simulink model "gm_nrhdlSignalDetection"  (R2023b)
settings: Solver=FixedStepDiscrete  StartTime=0.0  StopTime=sl_in.stopTime  RelTol=1e-3
undefined symbols (not defined in the file or in its folder): sl_in
libraries: hdlmdlgenlib x9, hdlsllib x5, simulink x4, dsphdlfiltering2 x4, dspsrcs4 x3, whdlmod x1
(part 1 of 2)
settings Model: SimulationMode=accelerator  Creator=The MathWorks, Inc.  LastModifiedBy=kgonipati
settings OptimizationCC: BlockReduction=off  ConditionallyExecuteInputs=off  DefaultParameterBehavior=Inlined  InheritOutputTypeSmallerThanSingle=on  ReuseModelBlockBuffer=off
settings DebuggingCC: AlgebraicLoopMsg=error  InheritedTsInSrcMsg=none  SingleTaskRateTransMsg=error  SubsystemReferenceDiagnosticForUnitTest=warning
settings HardwareCC: ProdBitPerPointer=32  ProdBitPerSizeT=32  ProdBitPerPtrDiffT=32  ProdLargestAtomicFloat=None  ProdIntDivRoundTo=Undefined  ProdEndianess=Unspecified  ProdWordSize=32  ProdHWDeviceType=ASIC/FPGA->ASIC/FPGA  TargetBitPerPointer=64  TargetBitPerSizeT=64  TargetBitPerPtrDiffT=64  TargetLongLongMode=on  TargetIntDivRoundTo=Zero  TargetEndianess=LittleEndian  TargetWordSize=64  TargetHWDeviceType=Custom Processor->MATLAB Host Computer  ProdEqTarget=off

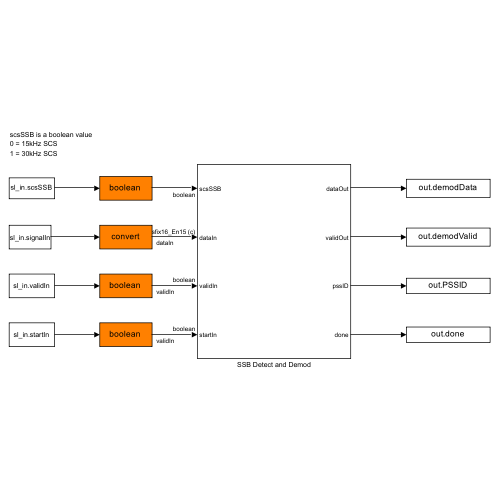
[thumbnail: Simulink's stored preview of the top-level diagram]
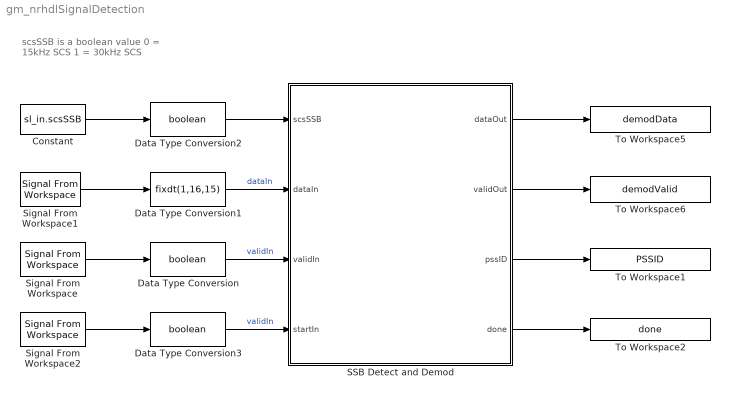
== system gm_nrhdlSignalDetection ==
  note: scsSSB is a boolean value
      | 0 = 15kHz SCS
      | 1 = 30kHz SCS
  Constant : Constant  Value=sl_in.scsSSB  SampleTime=sl_in.sampleTime
  Data Type Conversion : DataTypeConversion  OutDataTypeStr=boolean  SaturateOnIntegerOverflow=off  RndMeth=Floor
  Data Type Conversion1 : DataTypeConversion  OutDataTypeStr=fixdt(1,16,15)  RndMeth=Round  SaturateOnIntegerOverflow=off
  Data Type Conversion2 : DataTypeConversion  OutDataTypeStr=boolean  SaturateOnIntegerOverflow=off  RndMeth=Floor
  Data Type Conversion3 : DataTypeConversion  OutDataTypeStr=boolean  SaturateOnIntegerOverflow=off  RndMeth=Floor
  SSB Detect and Demod : Subsystem
  Signal From Workspace : dspsrcs4/Signal From Workspace  X=sl_in.validIn  Ts=sl_in.sampleTime  nsamps=1  OutputAfterFinalValue=Setting to zero  ignoreOrWarnInputAndFrameLengths=off  OutputFrames=off
  Signal From Workspace1 : dspsrcs4/Signal From Workspace  X=sl_in.signalIn  Ts=sl_in.sampleTime  nsamps=1  OutputAfterFinalValue=Setting to zero  ignoreOrWarnInputAndFrameLengths=off  OutputFrames=off
  Signal From Workspace2 : dspsrcs4/Signal From Workspace  X=sl_in.startIn  Ts=sl_in.sampleTime  nsamps=1  OutputAfterFinalValue=Setting to zero  ignoreOrWarnInputAndFrameLengths=off  OutputFrames=off
  To Workspace1 : ToWorkspace  VariableName=PSSID  SampleTime=-1
      settings: Save2DSignal=2-D array (concatenate along first dimension)
  To Workspace2 : ToWorkspace  VariableName=done  SampleTime=-1
      settings: Save2DSignal=2-D array (concatenate along first dimension)
  To Workspace5 : ToWorkspace  VariableName=demodData  SampleTime=-1
      settings: Save2DSignal=2-D array (concatenate along first dimension)
  To Workspace6 : ToWorkspace  VariableName=demodValid  SampleTime=-1
      settings: Save2DSignal=2-D array (concatenate along first dimension)
  wires:
  SSB Detect and Demod/4(done) -> To Workspace2/1
  Data Type Conversion3/1 -> SSB Detect and Demod/4(startIn)  "validIn"
  Signal From Workspace2/1 -> Data Type Conversion3/1
  Data Type Conversion2/1 -> SSB Detect and Demod/1(scsSSB)
  SSB Detect and Demod/3(pssID) -> To Workspace1/1
  Constant/1 -> Data Type Conversion2/1
  Data Type Conversion1/1 -> SSB Detect and Demod/2(dataIn)  "dataIn"
  SSB Detect and Demod/2(validOut) -> To Workspace6/1
  SSB Detect and Demod/1(dataOut) -> To Workspace5/1
  Data Type Conversion/1 -> SSB Detect and Demod/3(validIn)  "validIn"
  Signal From Workspace/1 -> Data Type Conversion/1
  Signal From Workspace1/1 -> Data Type Conversion1/1

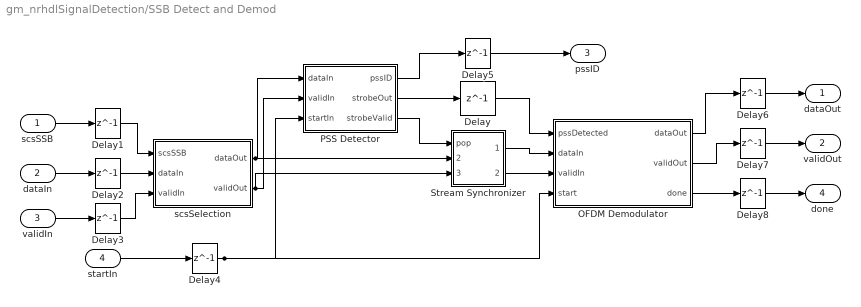
== system gm_nrhdlSignalDetection/SSB Detect and Demod ==
  scsSSB : Inport  OutDataTypeStr=boolean  PortDimensions=1  SampleTime=1.62760416666667e-08
  dataIn : Inport  Port=2  OutDataTypeStr=fixdt(1, 16, 15)  PortDimensions=1  SampleTime=1.62760416666667e-08
      settings: SignalType=complex
  validIn : Inport  Port=3  OutDataTypeStr=boolean  PortDimensions=1  SampleTime=1.62760416666667e-08
  startIn : Inport  Port=4  OutDataTypeStr=boolean  PortDimensions=1  SampleTime=1.62760416666667e-08
  Delay{,1..8} (9 alike) : Delay  DelayLength=1
  OFDM Demodulator : Subsystem
  PSS Detector : Subsystem
  Stream Synchronizer : Subsystem  mask{depth=double(512)}
  scsSelection : Subsystem
  dataOut : Outport  SampleTime=1.62760416666667e-08
  validOut : Outport  Port=2  SampleTime=1.62760416666667e-08
  pssID : Outport  Port=3  SampleTime=1.62760416666667e-08
  done : Outport  Port=4  SampleTime=1.62760416666667e-08
  wires:
  Delay1/1 -> scsSelection/1(scsSSB)
  scsSSB/1 -> Delay1/1
  Delay2/1 -> scsSelection/2(dataIn)
  dataIn/1 -> Delay2/1
  Delay3/1 -> scsSelection/3(validIn)
  validIn/1 -> Delay3/1
  scsSelection/1(dataOut) -> Stream Synchronizer/2(dataIn), PSS Detector/1(dataIn)
  startIn/1 -> Delay4/1
  scsSelection/2(validOut) -> Stream Synchronizer/3(push), PSS Detector/2(validIn)
  Delay4/1 -> OFDM Demodulator/4(start), PSS Detector/3(startIn)
  PSS Detector/1(pssID) -> Delay5/1
  PSS Detector/2(strobeOut) -> Delay/1
  PSS Detector/3(strobeValid) -> Stream Synchronizer/1(pop)
  Delay5/1 -> pssID/1
  Delay/1 -> OFDM Demodulator/1(pssDetected)
  Stream Synchronizer/2(validOut) -> OFDM Demodulator/3(validIn)
  Stream Synchronizer/1(dataOut) -> OFDM Demodulator/2(dataIn)
  OFDM Demodulator/1(dataOut) -> Delay6/1
  OFDM Demodulator/2(validOut) -> Delay7/1
  OFDM Demodulator/3(done) -> Delay8/1
  Delay6/1 -> dataOut/1
  Delay7/1 -> validOut/1
  Delay8/1 -> done/1

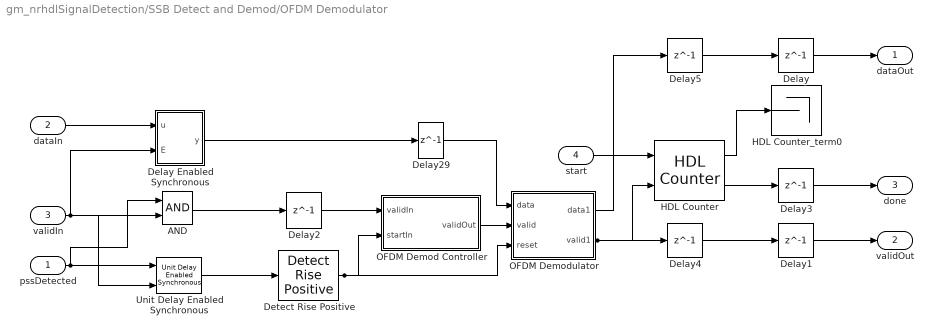
== system gm_nrhdlSignalDetection/SSB Detect and Demod/OFDM Demodulator ==
  pssDetected : Inport  OutDataTypeStr=boolean  PortDimensions=1  SampleTime=1.62760416666667e-08
  dataIn : Inport  Port=2  OutDataTypeStr=fixdt(1, 16, 15)  PortDimensions=1  SampleTime=1.62760416666667e-08
      settings: SignalType=complex
  validIn : Inport  Port=3  OutDataTypeStr=boolean  PortDimensions=1  SampleTime=1.62760416666667e-08
  start : Inport  Port=4  OutDataTypeStr=boolean  PortDimensions=1  SampleTime=1.62760416666667e-08
  AND : Logic  AllPortsSameDT=off  OutDataTypeStr=boolean
  Delay{,1..5,29} (7 alike) : Delay  DelayLength=1
  Delay Enabled Synchronous : Subsystem  mask(Delay Enabled){DelayLength=256+18, InitialCondition=0.0}
      mask prompts: DelayLength "Simulink:blkprm_prompts:DelayBlkDelayLength"; InitialCondition "Simulink:blkprm_prompts:DelayBlkInitCond"
      mask help: Implements a delay with synchronous enable.
      mask Display:
      | port_label('input', 1, 'u');
      | port_label('input', 2, 'E');
      | text(0.45,0.45, 'Z');
      | DelayLengthStr = get_param(gcbh,'DelayLength');
      | try
      |     DelayLength = eval(DelayLengthStr);
      |     text(0.55,0.55, sprintf('-%d',DelayLength));
      | catch ME
      |     text(0.55,0.55, '-N');
      | end
  Detect Rise Positive : simulink/Logic and Bit Operations/Detect Rise Positive  vinit=0  OutDataTypeStr=boolean
  HDL Counter : hdlsllib/Sources/HDL Counter  CountType=Count limited  CountInit=0  CountStep=1  CountMax=960  CountFromType=Initial value  CountFrom=0  CountResetPort=on  CountLoadPort=off  CountEnbPort=on  CountDirPort=off  CountHitOutputPort=on  CountDataType=Unsigned  CountWordLen=12  CountFracLen=0  CountSampTime=1
  HDL Counter_term0 : Terminator
  OFDM Demod Controller : Subsystem
  OFDM Demodulator : Subsystem
  Unit Delay Enabled Synchronous : hdlsllib/Discrete/Unit Delay Enabled Synchronous  InitialCondition=0.0  SampleTime=-1
  dataOut : Outport  SampleTime=1.62760416666667e-08
  validOut : Outport  Port=2  SampleTime=1.62760416666667e-08
  done : Outport  Port=3  SampleTime=1.62760416666667e-08
  wires:
  Detect Rise Positive/1 -> OFDM Demodulator/3(reset), OFDM Demod Controller/2(startIn)
  dataIn/1 -> Delay Enabled Synchronous/1(u)
  pssDetected/1 -> AND/1, Unit Delay Enabled Synchronous/1
  Delay Enabled Synchronous/1(y) -> Delay29/1
  validIn/1 -> AND/2, Delay Enabled Synchronous/2(E), Unit Delay Enabled Synchronous/2
  AND/1 -> Delay2/1
  Delay2/1 -> OFDM Demod Controller/1(validIn)
  Delay5/1 -> Delay/1
  Unit Delay Enabled Synchronous/1 -> Detect Rise Positive/1
  Delay29/1 -> OFDM Demodulator/1(data)
  OFDM Demod Controller/1(validOut) -> OFDM Demodulator/2(valid)
  start/1 -> HDL Counter/1
  Delay/1 -> dataOut/1
  OFDM Demodulator/1(data1) -> Delay5/1
  OFDM Demodulator/2(valid1) -> Delay4/1, HDL Counter/2
  HDL Counter/1 -> HDL Counter_term0/1
  HDL Counter/2 -> Delay3/1
  Delay1/1 -> validOut/1
  Delay4/1 -> Delay1/1
  Delay3/1 -> done/1

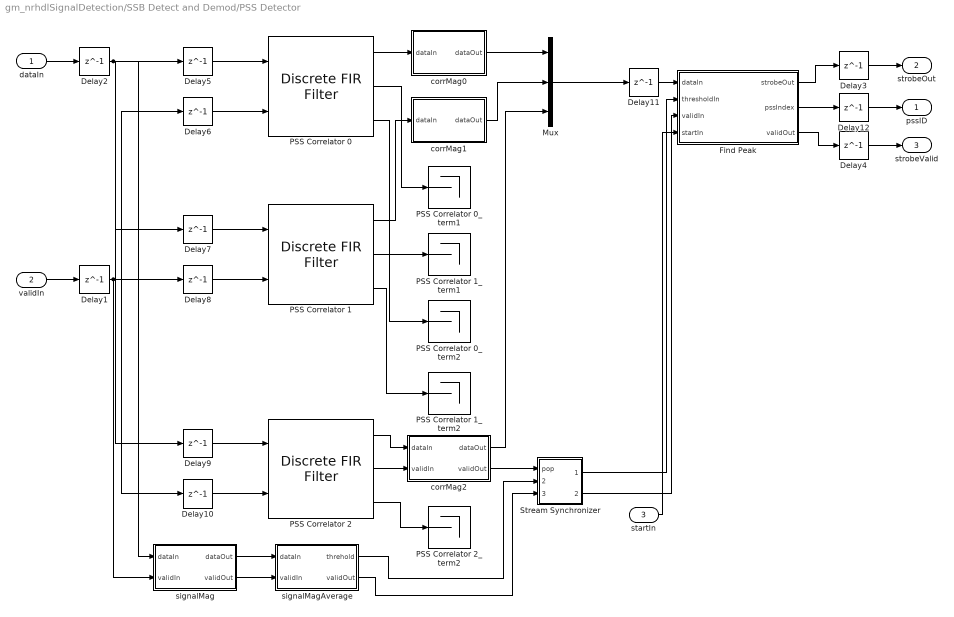
== system gm_nrhdlSignalDetection/SSB Detect and Demod/PSS Detector ==
  dataIn : Inport  OutDataTypeStr=fixdt(1, 16, 15)  PortDimensions=1  SampleTime=1.62760416666667e-08
      settings: SignalType=complex
  validIn : Inport  Port=2  OutDataTypeStr=boolean  PortDimensions=1  SampleTime=1.62760416666667e-08
  startIn : Inport  Port=3  OutDataTypeStr=boolean  PortDimensions=1  SampleTime=1.62760416666667e-08
  Delay{1..12} (12 alike) : Delay  DelayLength=1
  Find Peak : Subsystem
  Mux : Mux  Inputs=3
  PSS Correlator 0 : dsphdlfiltering2/Discrete FIR Filter  NumeratorSource=Property  Numerator=sl_in.pssCorrelationCoeffs(:,1).'  NumeratorPrototype=[]  FilterStructure=Partly serial systolic  SerializationOption=Minimum number of cycles between valid input samples  NumCycles=sl_in.cyclesPerSample  NumberOfMultipliers=2  SimulateUsing=Code generation  roundingMode=Floor  overflowMode=off  CoefficientsDataTypeStr=fixdt(1,8,10)  OutputDataTypeStr=fixdt(1,18,13)  ResetInputPort=off  HDLGlobalReset=off  CoeffMultiplier=Multiplier  UseMultForPow2Coeff=on
  PSS Correlator 0_term1 : Terminator
  PSS Correlator 0_term2 : Terminator
  PSS Correlator 1 : dsphdlfiltering2/Discrete FIR Filter  NumeratorSource=Property  Numerator=sl_in.pssCorrelationCoeffs(:,2).'  NumeratorPrototype=[]  FilterStructure=Partly serial systolic  SerializationOption=Minimum number of cycles between valid input samples  NumCycles=sl_in.cyclesPerSample  NumberOfMultipliers=2  SimulateUsing=Code generation  roundingMode=Floor  overflowMode=off  CoefficientsDataTypeStr=fixdt(1,8,10)  OutputDataTypeStr=fixdt(1,18,13)  ResetInputPort=off  HDLGlobalReset=off  CoeffMultiplier=Multiplier  UseMultForPow2Coeff=on
  PSS Correlator 1_term1 : Terminator
  PSS Correlator 1_term2 : Terminator
  PSS Correlator 2 : dsphdlfiltering2/Discrete FIR Filter  NumeratorSource=Property  Numerator=sl_in.pssCorrelationCoeffs(:,3).'  NumeratorPrototype=[]  FilterStructure=Partly serial systolic  SerializationOption=Minimum number of cycles between valid input samples  NumCycles=sl_in.cyclesPerSample  NumberOfMultipliers=2  SimulateUsing=Code generation  roundingMode=Floor  overflowMode=off  CoefficientsDataTypeStr=fixdt(1,8,10)  OutputDataTypeStr=fixdt(1,18,13)  ResetInputPort=off  HDLGlobalReset=off  CoeffMultiplier=Multiplier  UseMultForPow2Coeff=on
  PSS Correlator 2_term2 : Terminator
  Stream Synchronizer : Subsystem  mask{depth=double(512)}
  corrMag0 : Subsystem
  corrMag1 : Subsystem
  corrMag2 : Subsystem
  signalMag : Subsystem
  signalMagAverage : Subsystem
  pssID : Outport  SampleTime=1.62760416666667e-08
  strobeOut : Outport  Port=2  SampleTime=1.62760416666667e-08
  strobeValid : Outport  Port=3  SampleTime=1.62760416666667e-08
  wires:
  Delay8/1 -> PSS Correlator 1/2
  dataIn/1 -> Delay2/1
  startIn/1 -> Find Peak/4(startIn)
  validIn/1 -> Delay1/1
  PSS Correlator 2/2 -> corrMag2/2(validIn)
  Delay2/1 -> Delay7/1, signalMag/1(dataIn), Delay5/1, Delay9/1
  Delay1/1 -> Delay6/1, Delay10/1, Delay8/1, signalMag/2(validIn)
  Delay5/1 -> PSS Correlator 0/1
  Stream Synchronizer/1(dataOut) -> Find Peak/2(thresholdIn)
  Delay6/1 -> PSS Correlator 0/2
  corrMag0/1(dataOut) -> Mux/1
  Delay7/1 -> PSS Correlator 1/1
  Delay9/1 -> PSS Correlator 2/1
  Delay10/1 -> PSS Correlator 2/2
  signalMag/2(validOut) -> signalMagAverage/2(validIn)
  signalMag/1(dataOut) -> signalMagAverage/1(dataIn)
  PSS Correlator 0/2 -> PSS Correlator 0_term1/1
  PSS Correlator 0/1 -> corrMag0/1(dataIn)
  PSS Correlator 0/3 -> PSS Correlator 0_term2/1
  PSS Correlator 1/1 -> corrMag1/1(dataIn)
  Delay11/1 -> Find Peak/1(dataIn)
  PSS Correlator 1/3 -> PSS Correlator 1_term2/1
  PSS Correlator 1/2 -> PSS Correlator 1_term1/1
  PSS Correlator 2/1 -> corrMag2/1(dataIn)
  PSS Correlator 2/3 -> PSS Correlator 2_term2/1
  signalMagAverage/1(threhold) -> Stream Synchronizer/2(dataIn)
  signalMagAverage/2(validOut) -> Stream Synchronizer/3(push)
  corrMag1/1(dataOut) -> Mux/2
  corrMag2/2(validOut) -> Stream Synchronizer/1(pop)
  corrMag2/1(dataOut) -> Mux/3
  Mux/1 -> Delay11/1
  Stream Synchronizer/2(validOut) -> Find Peak/3(validIn)
  Find Peak/1(strobeOut) -> Delay3/1
  Find Peak/2(pssIndex) -> Delay12/1
  Find Peak/3(validOut) -> Delay4/1
  Delay4/1 -> strobeValid/1
  Delay3/1 -> strobeOut/1
  Delay12/1 -> pssID/1

== system gm_nrhdlSignalDetection/SSB Detect and Demod/Stream Synchronizer ==
  pop : Inport  OutDataTypeStr=boolean  PortDimensions=1  SampleTime=1.62760416666667e-08
  dataIn : Inport  Port=2  OutDataTypeStr=fixdt(1, 16, 15)  PortDimensions=1  SampleTime=1.62760416666667e-08
      settings: SignalType=complex
  push : Inport  Port=3  OutDataTypeStr=boolean  PortDimensions=1  SampleTime=1.62760416666667e-08
  MATLAB Function : Subsystem
  Simple Dual Port RAM System : hdlsllib/HDL RAMs/Simple Dual Port RAM System  RAMType=Simple dual port  AsyncRead=off  WriteOutputValue=New data  RAMInitialValue=0  allowBusInputs=off  WritesHaveOutput=on  NumReads=0  NumWrites=1  SimulateUsing=Code generation
  dataOut : Outport  SampleTime=1.62760416666667e-08
  validOut : Outport  Port=2  SampleTime=1.62760416666667e-08
  wires:
  pop/1 -> MATLAB Function/1(pop)
  dataIn/1 -> Simple Dual Port RAM System/1
  push/1 -> MATLAB Function/2(push)
  MATLAB Function/1(wrAddr) -> Simple Dual Port RAM System/2
  Simple Dual Port RAM System/1 -> dataOut/1
  MATLAB Function/2(wrEn) -> Simple Dual Port RAM System/3
  MATLAB Function/3(rdAddr) -> Simple Dual Port RAM System/4
  MATLAB Function/4(validOut) -> validOut/1

== system gm_nrhdlSignalDetection/SSB Detect and Demod/scsSelection ==
  note: Decimate to 15KHz SCS rate
  scsSSB : Inport  OutDataTypeStr=boolean  PortDimensions=1  SampleTime=1.62760416666667e-08
  dataIn : Inport  Port=2  OutDataTypeStr=fixdt(1, 16, 15)  PortDimensions=1  SampleTime=1.62760416666667e-08
      settings: SignalType=complex
  validIn : Inport  Port=3  OutDataTypeStr=boolean  PortDimensions=1  SampleTime=1.62760416666667e-08
  Data Type Conversion : DataTypeConversion  OutDataTypeStr=fixdt(1,16,15)  RndMeth=Round  SaturateOnIntegerOverflow=off
  FIR Decimator : dsphdlfiltering2/FIR Decimator  Numerator=sl_in.halfbandCoeffs  FilterStructure=Direct form systolic  DecimationFactor=2  NumCycles=sl_in.cyclesPerSample  SimulateUsing=Code generation  roundingMode=Round  overflowMode=off  CoefficientsDataTypeStr=fixdt(1,16,16)  ResetInputPort=off  HDLGlobalReset=off
  Multiport Switch : MultiPortSwitch  DataPortOrder=Zero-based contiguous  Inputs=2  zeroidx=on  SaturateOnIntegerOverflow=off  InputSameDT=off
  Multiport Switch1 : MultiPortSwitch  DataPortOrder=Zero-based contiguous  Inputs=2  zeroidx=on  SaturateOnIntegerOverflow=off  InputSameDT=off
  Transient Removal : Subsystem
  dataOut : Outport  SampleTime=1.62760416666667e-08
  validOut : Outport  Port=2  SampleTime=1.62760416666667e-08
  wires:
  Transient Removal/1(dataOut) -> Multiport Switch/2
  FIR Decimator/1 -> Data Type Conversion/1
  dataIn/1 -> Multiport Switch/3, FIR Decimator/1
  validIn/1 -> Multiport Switch1/3, FIR Decimator/2
  Transient Removal/2(validOut) -> Multiport Switch1/2
  FIR Decimator/2 -> Transient Removal/2(validIn)
  Data Type Conversion/1 -> Transient Removal/1(dataIn)
  scsSSB/1 -> Multiport Switch1/1, Multiport Switch/1
  Multiport Switch/1 -> dataOut/1
  Multiport Switch1/1 -> validOut/1

== system gm_nrhdlSignalDetection/SSB Detect and Demod/OFDM Demodulator/Delay Enabled Synchronous ==
  u : Inport  OutDataTypeStr=fixdt(1, 16, 15)  PortDimensions=1  SampleTime=1.62760416666667e-08
      settings: SignalType=complex
  E : Inport  Port=2  OutDataTypeStr=boolean  PortDimensions=1  SampleTime=1.62760416666667e-08
  Synchronous Delay : Subsystem
  y : Outport  SampleTime=1.62760416666667e-08
  wires:
  u/1 -> Synchronous Delay/1(u)
  E/1 -> Synchronous Delay/2(E)
  Synchronous Delay/1(y) -> y/1

== system gm_nrhdlSignalDetection/SSB Detect and Demod/OFDM Demodulator/OFDM Demod Controller ==
  validIn : Inport  OutDataTypeStr=boolean  PortDimensions=1  SampleTime=1.62760416666667e-08
  startIn : Inport  Port=2  OutDataTypeStr=boolean  PortDimensions=1  SampleTime=1.62760416666667e-08
  OFDM Demod Controller : MATLAB Function  TreatAsAtomicUnit=on
  OFDM Demod Controller_term1 : Terminator
  validOut : Outport  SampleTime=1.62760416666667e-08
  wires:
  OFDM Demod Controller/1(validOut) -> validOut/1
  validIn/1 -> OFDM Demod Controller/1(validIn)
  OFDM Demod Controller/2(done) -> OFDM Demod Controller_term1/1
  startIn/1 -> OFDM Demod Controller/2(startIn)

== system gm_nrhdlSignalDetection/SSB Detect and Demod/OFDM Demodulator/OFDM Demodulator ==
  data : Inport  OutDataTypeStr=fixdt(1, 16, 15)  SampleTime=1.62760416666667e-08
      settings: SignalType=complex
  valid : Inport  Port=2  OutDataTypeStr=boolean  SampleTime=1.62760416666667e-08
  reset : Inport  Port=3  OutDataTypeStr=boolean  SampleTime=1.62760416666667e-08
  OFDM Demodulator : whdlmod/OFDM Demodulator  OFDMParamsSource=Property  MaxFFTLength=256  FFTLength=256  CPLength=18  NumLGsC=8  NumRGsC=8  CPFraction=on  CPFractionSource=Property  CPFractionValue=0.5  removeDCSubcarriers=off  enableResetInputPort=on  Normalize=off  RoundingMethod=Round  SimulateUsing=Code generation
  data1 : Outport  SampleTime=1.62760416666667e-08
  valid1 : Outport  Port=2  SampleTime=1.62760416666667e-08
  wires:
  data/1 -> OFDM Demodulator/1
  valid/1 -> OFDM Demodulator/2
  OFDM Demodulator/1 -> data1/1
  reset/1 -> OFDM Demodulator/3
  OFDM Demodulator/2 -> valid1/1

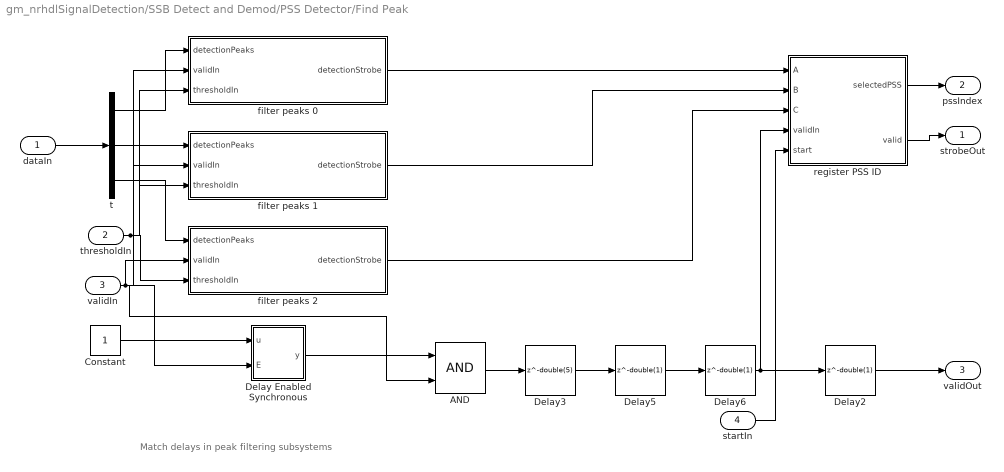
== system gm_nrhdlSignalDetection/SSB Detect and Demod/PSS Detector/Find Peak ==
  note: Match delays in peak filtering subsystems
  dataIn : Inport  OutDataTypeStr=fixdt(1, 36, 26)  PortDimensions=[3]  SampleTime=1.62760416666667e-08
  thresholdIn : Inport  Port=2  OutDataTypeStr=fixdt(0, 32, 24)  PortDimensions=1  SampleTime=1.62760416666667e-08
  validIn : Inport  Port=3  OutDataTypeStr=boolean  PortDimensions=1  SampleTime=1.62760416666667e-08
  startIn : Inport  Port=4  OutDataTypeStr=boolean  PortDimensions=1  SampleTime=1.62760416666667e-08
  AND : Logic  AllPortsSameDT=off  OutDataTypeStr=boolean  SampleTime=1.62760416666667e-08
  Constant : Constant  OutDataTypeStr=boolean  SampleTime=1.62760416666667e-08
  Delay Enabled Synchronous : Subsystem  mask(Delay Enabled){DelayLength=ceil(sl_in.windowLength/2), InitialCondition=0.0}
      mask prompts: DelayLength "Simulink:blkprm_prompts:DelayBlkDelayLength"; InitialCondition "Simulink:blkprm_prompts:DelayBlkInitCond"
      mask help: Implements a delay with synchronous enable.
      mask Display:
      | port_label('input', 1, 'u');
      | port_label('input', 2, 'E');
      | text(0.45,0.45, 'Z');
      | DelayLengthStr = get_param(gcbh,'DelayLength');
      | try
      |     DelayLength = eval(DelayLengthStr);
      |     text(0.55,0.55, sprintf('-%d',DelayLength));
      | catch ME
      |     text(0.55,0.55, '-N');
      | end
  Delay2 : Delay  DelayLength=double(1)  InitialCondition=0  SampleTime=1.62760416666667e-08
  Delay3 : Delay  DelayLength=double(5)  InitialCondition=0  SampleTime=1.62760416666667e-08
  Delay5 : Delay  DelayLength=double(1)  InitialCondition=0  SampleTime=1.62760416666667e-08
  Delay6 : Delay  DelayLength=double(1)  InitialCondition=0  SampleTime=1.62760416666667e-08
  filter peaks 0 : Subsystem
  filter peaks 1 : Subsystem
  filter peaks 2 : Subsystem
  register PSS ID : Subsystem
  t : Demux  Outputs=3
  strobeOut : Outport  SampleTime=1.62760416666667e-08
  pssIndex : Outport  Port=2  SampleTime=1.62760416666667e-08
  validOut : Outport  Port=3  SampleTime=1.62760416666667e-08
  wires:
  t/3 -> filter peaks 2/1(detectionPeaks)
  dataIn/1 -> t/1
  validIn/1 -> AND/2, filter peaks 2/2(validIn), filter peaks 0/2(validIn), filter peaks 1/2(validIn), Delay Enabled Synchronous/2(E)
  t/1 -> filter peaks 0/1(detectionPeaks)
  thresholdIn/1 -> filter peaks 2/3(thresholdIn), filter peaks 0/3(thresholdIn), filter peaks 1/3(thresholdIn)
  t/2 -> filter peaks 1/1(detectionPeaks)
  Constant/1 -> Delay Enabled Synchronous/1(u)
  filter peaks 0/1(detectionStrobe) -> register PSS ID/1(A)
  filter peaks 1/1(detectionStrobe) -> register PSS ID/2(B)
  filter peaks 2/1(detectionStrobe) -> register PSS ID/3(C)
  Delay Enabled Synchronous/1(y) -> AND/1
  AND/1 -> Delay3/1
  Delay3/1 -> Delay5/1
  Delay5/1 -> Delay6/1
  Delay6/1 -> Delay2/1, register PSS ID/4(validIn)
  Delay2/1 -> validOut/1
  startIn/1 -> register PSS ID/5(start)
  register PSS ID/2(valid) -> strobeOut/1
  register PSS ID/1(selectedPSS) -> pssIndex/1

== system gm_nrhdlSignalDetection/SSB Detect and Demod/PSS Detector/Stream Synchronizer ==
  pop : Inport  OutDataTypeStr=boolean  PortDimensions=1  SampleTime=1.62760416666667e-08
  dataIn : Inport  Port=2  OutDataTypeStr=fixdt(0, 32, 24)  PortDimensions=1  SampleTime=1.62760416666667e-08
  push : Inport  Port=3  OutDataTypeStr=boolean  PortDimensions=1  SampleTime=1.62760416666667e-08
  MATLAB Function : Subsystem
  Simple Dual Port RAM System : hdlsllib/HDL RAMs/Simple Dual Port RAM System  RAMType=Simple dual port  AsyncRead=off  WriteOutputValue=New data  RAMInitialValue=0  allowBusInputs=off  WritesHaveOutput=on  NumReads=0  NumWrites=1  SimulateUsing=Code generation
  dataOut : Outport  SampleTime=1.62760416666667e-08
  validOut : Outport  Port=2  SampleTime=1.62760416666667e-08
  wires:
  pop/1 -> MATLAB Function/1(pop)
  dataIn/1 -> Simple Dual Port RAM System/1
  push/1 -> MATLAB Function/2(push)
  MATLAB Function/1(wrAddr) -> Simple Dual Port RAM System/2
  MATLAB Function/3(rdAddr) -> Simple Dual Port RAM System/4
  MATLAB Function/2(wrEn) -> Simple Dual Port RAM System/3
  MATLAB Function/4(validOut) -> validOut/1
  Simple Dual Port RAM System/1 -> dataOut/1

== system gm_nrhdlSignalDetection/SSB Detect and Demod/PSS Detector/corrMag0 ==
  dataIn : Inport  OutDataTypeStr=fixdt(1, 18, 13)  PortDimensions=1  SampleTime=1.62760416666667e-08
      settings: SignalType=complex
  Add : Sum  OutDataTypeStr=Inherit: Same as accumulator
  Complex to Real-Imag : ComplexToRealImag
  Delay{2..6} (5 alike) : Delay  DelayLength=1
  Product : Product
  Product1 : Product
  dataOut : Outport  SampleTime=1.62760416666667e-08
  wires:
  Complex to Real-Imag/2 -> Delay3/1
  dataIn/1 -> Complex to Real-Imag/1
  Complex to Real-Imag/1 -> Delay2/1
  Delay2/1 -> Product/2, Product/1
  Delay3/1 -> Product1/1, Product1/2
  Product1/1 -> Delay5/1
  Product/1 -> Delay4/1
  Delay4/1 -> Add/1
  Delay5/1 -> Add/2
  Add/1 -> Delay6/1
  Delay6/1 -> dataOut/1

== system gm_nrhdlSignalDetection/SSB Detect and Demod/PSS Detector/corrMag1 ==
  dataIn : Inport  OutDataTypeStr=fixdt(1, 18, 13)  PortDimensions=1  SampleTime=1.62760416666667e-08
      settings: SignalType=complex
  Add : Sum  OutDataTypeStr=Inherit: Same as accumulator
  Complex to Real-Imag : ComplexToRealImag
  Delay{2..6} (5 alike) : Delay  DelayLength=1
  Product : Product
  Product1 : Product
  dataOut : Outport  SampleTime=1.62760416666667e-08
  wires:
  dataIn/1 -> Complex to Real-Imag/1
  Complex to Real-Imag/1 -> Delay2/1
  Complex to Real-Imag/2 -> Delay3/1
  Delay2/1 -> Product/2, Product/1
  Delay3/1 -> Product1/2, Product1/1
  Product/1 -> Delay4/1
  Product1/1 -> Delay5/1
  Delay4/1 -> Add/1
  Delay5/1 -> Add/2
  Add/1 -> Delay6/1
  Delay6/1 -> dataOut/1

== system gm_nrhdlSignalDetection/SSB Detect and Demod/PSS Detector/corrMag2 ==
  dataIn : Inport  OutDataTypeStr=fixdt(1, 18, 13)  PortDimensions=1  SampleTime=1.62760416666667e-08
      settings: SignalType=complex
  validIn : Inport  Port=2  OutDataTypeStr=boolean  PortDimensions=1  SampleTime=1.62760416666667e-08
  Add : Sum  OutDataTypeStr=Inherit: Same as accumulator
  Complex to Real-Imag : ComplexToRealImag
  Delay{2..9} (8 alike) : Delay  DelayLength=1
  Product : Product
  Product1 : Product
  dataOut : Outport  SampleTime=1.62760416666667e-08
  validOut : Outport  Port=2  SampleTime=1.62760416666667e-08
  wires:
  validIn/1 -> Delay7/1
  Complex to Real-Imag/2 -> Delay3/1
  dataIn/1 -> Complex to Real-Imag/1
  Delay7/1 -> Delay8/1
  Delay3/1 -> Product1/2, Product1/1
  Delay8/1 -> Delay9/1
  Complex to Real-Imag/1 -> Delay2/1
  Delay2/1 -> Product/2, Product/1
  Delay9/1 -> validOut/1
  Product/1 -> Delay4/1
  Product1/1 -> Delay5/1
  Delay4/1 -> Add/1
  Delay5/1 -> Add/2
  Add/1 -> Delay6/1
  Delay6/1 -> dataOut/1

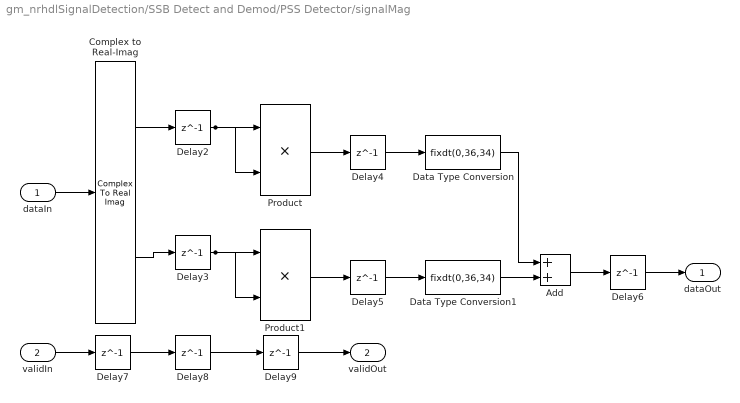
== system gm_nrhdlSignalDetection/SSB Detect and Demod/PSS Detector/signalMag ==
  dataIn : Inport  OutDataTypeStr=fixdt(1, 16, 15)  PortDimensions=1  SampleTime=1.62760416666667e-08
      settings: SignalType=complex
  validIn : Inport  Port=2  OutDataTypeStr=boolean  PortDimensions=1  SampleTime=1.62760416666667e-08
  Add : Sum
  Complex to Real-Imag : ComplexToRealImag
  Data Type Conversion : DataTypeConversion  OutDataTypeStr=fixdt(0,36,34)  SaturateOnIntegerOverflow=off  RndMeth=Floor
  Data Type Conversion1 : DataTypeConversion  OutDataTypeStr=fixdt(0,36,34)  SaturateOnIntegerOverflow=off  RndMeth=Floor
  Delay{2..9} (8 alike) : Delay  DelayLength=1
  Product : Product
  Product1 : Product
  dataOut : Outport  SampleTime=1.62760416666667e-08
  validOut : Outport  Port=2  SampleTime=1.62760416666667e-08
  wires:
  dataIn/1 -> Complex to Real-Imag/1
  validIn/1 -> Delay7/1
  Delay8/1 -> Delay9/1
  Complex to Real-Imag/1 -> Delay2/1
  Delay3/1 -> Product1/2, Product1/1
  Complex to Real-Imag/2 -> Delay3/1
  Delay2/1 -> Product/2, Product/1
  Delay7/1 -> Delay8/1
  Product/1 -> Delay4/1
  Product1/1 -> Delay5/1
  Delay9/1 -> validOut/1
  Delay4/1 -> Data Type Conversion/1
  Delay5/1 -> Data Type Conversion1/1
  Data Type Conversion/1 -> Add/1
  Data Type Conversion1/1 -> Add/2
  Add/1 -> Delay6/1
  Delay6/1 -> dataOut/1

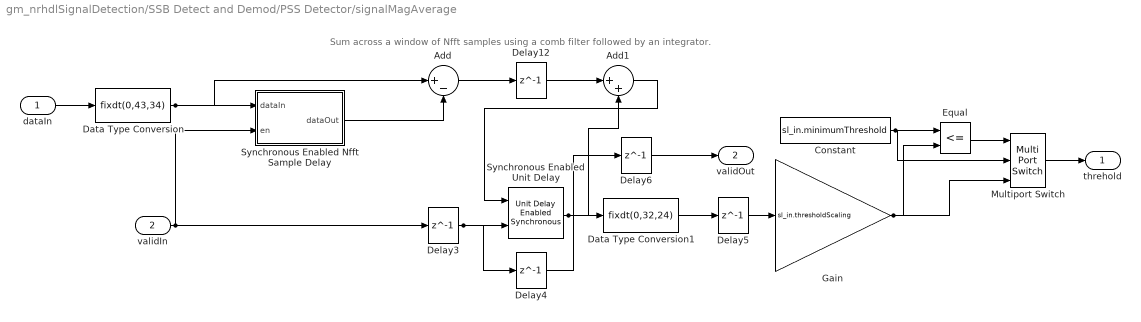
== system gm_nrhdlSignalDetection/SSB Detect and Demod/PSS Detector/signalMagAverage ==
  note: Sum across a window of Nfft samples using a comb filter followed by an integrator.
  dataIn : Inport  OutDataTypeStr=fixdt(0, 37, 34)  PortDimensions=1  SampleTime=1.62760416666667e-08
  validIn : Inport  Port=2  OutDataTypeStr=boolean  PortDimensions=1  SampleTime=1.62760416666667e-08
  Add : Sum  Inputs=|+-  OutDataTypeStr=Inherit: Same as accumulator
  Add1 : Sum  Inputs=|++  OutDataTypeStr=Inherit: Same as accumulator
  Constant : Constant  Value=sl_in.minimumThreshold  SampleTime=-1
  Data Type Conversion : DataTypeConversion  OutDataTypeStr=fixdt(0,43,34)  SaturateOnIntegerOverflow=off  RndMeth=Floor
  Data Type Conversion1 : DataTypeConversion  OutDataTypeStr=fixdt(0,32,24)  SaturateOnIntegerOverflow=off  RndMeth=Floor
  Delay{3..6,12} (5 alike) : Delay  DelayLength=1  InitialCondition=0
  Equal : RelationalOperator  Operator=<=  OutDataTypeStr=boolean  RndMeth=Simplest  InputSameDT=off
  Gain : Gain  Gain=sl_in.thresholdScaling  ParamDataTypeStr=Inherit: Inherit from 'Gain'  OutDataTypeStr=Inherit: Same as input
  Multiport Switch : MultiPortSwitch  DataPortOrder=Zero-based contiguous  Inputs=2  zeroidx=on  SaturateOnIntegerOverflow=off  InputSameDT=off
  "Synchronous Enabled Nfft Sample Delay " : Subsystem
  Synchronous Enabled Unit Delay : hdlsllib/Discrete/Unit Delay Enabled Synchronous  InitialCondition=0.0  SampleTime=-1
  threhold : Outport  SampleTime=1.62760416666667e-08  VectorParamsAs1DForOutWhenUnconnected=off
  validOut : Outport  Port=2  SampleTime=1.62760416666667e-08  VectorParamsAs1DForOutWhenUnconnected=off
  wires:
  "Synchronous Enabled Nfft Sample Delay "/1(dataOut) -> Add/2
  dataIn/1 -> Data Type Conversion/1
  validIn/1 -> Delay3/1, "Synchronous Enabled Nfft Sample Delay "/2(en)
  Data Type Conversion/1 -> Add/1, "Synchronous Enabled Nfft Sample Delay "/1(dataIn)
  Delay12/1 -> Add1/1
  Add/1 -> Delay12/1
  Delay3/1 -> Delay4/1, Synchronous Enabled Unit Delay/2
  Synchronous Enabled Unit Delay/1 -> Add1/2, Data Type Conversion1/1
  Delay4/1 -> Delay6/1
  Constant/1 -> Multiport Switch/2, Equal/1
  Add1/1 -> Synchronous Enabled Unit Delay/1
  Delay6/1 -> validOut/1
  Data Type Conversion1/1 -> Delay5/1
  Delay5/1 -> Gain/1
  Gain/1 -> Multiport Switch/3, Equal/2
  Equal/1 -> Multiport Switch/1
  Multiport Switch/1 -> threhold/1

== system gm_nrhdlSignalDetection/SSB Detect and Demod/Stream Synchronizer/MATLAB Function ==
  pop : Inport  OutDataTypeStr=boolean  PortDimensions=1  SampleTime=1.62760416666667e-08
  push : Inport  Port=2  OutDataTypeStr=boolean  PortDimensions=1  SampleTime=1.62760416666667e-08
  MATLAB Function : MATLAB Function  InitFcn=Simulink.suppressDiagnostic(gcb, 'Stateflow:Runtime:DataOverflowErrorMSLD');  TreatAsAtomicUnit=on
  wrAddr : Outport  SampleTime=1.62760416666667e-08
  wrEn : Outport  Port=2  SampleTime=1.62760416666667e-08
  rdAddr : Outport  Port=3  SampleTime=1.62760416666667e-08
  validOut : Outport  Port=4  SampleTime=1.62760416666667e-08
  wires:
  pop/1 -> MATLAB Function/1(pop)
  push/1 -> MATLAB Function/2(push)
  MATLAB Function/1(wrAddr) -> wrAddr/1
  MATLAB Function/2(wrEn) -> wrEn/1
  MATLAB Function/3(rdAddr) -> rdAddr/1
  MATLAB Function/4(validOut) -> validOut/1

== system gm_nrhdlSignalDetection/SSB Detect and Demod/scsSelection/Transient Removal ==
  dataIn : Inport  OutDataTypeStr=fixdt(1, 16, 15)  PortDimensions=1  SampleTime=1.62760416666667e-08
      settings: SignalType=complex
  validIn : Inport  Port=2  OutDataTypeStr=boolean  PortDimensions=1  SampleTime=1.62760416666667e-08
  Transient Removal : MATLAB Function  TreatAsAtomicUnit=on  mask{TransientLength=sl_in.halfbandTransient}
      mask prompts: TransientLength "Transient length"
  dataOut : Outport  SampleTime=1.62760416666667e-08  VectorParamsAs1DForOutWhenUnconnected=off
  validOut : Outport  Port=2  SampleTime=1.62760416666667e-08  VectorParamsAs1DForOutWhenUnconnected=off
  wires:
  dataIn/1 -> Transient Removal/1(dataIn)
  validIn/1 -> Transient Removal/2(validIn)
  Transient Removal/1(dataOut) -> dataOut/1
  Transient Removal/2(validOut) -> validOut/1

== system gm_nrhdlSignalDetection/SSB Detect and Demod/OFDM Demodulator/Delay Enabled Synchronous/Synchronous Delay ==
  u : Inport  OutDataTypeStr=fixdt(1, 16, 15)  PortDimensions=1  SampleTime=1.62760416666667e-08
      settings: SignalType=complex
  E : Inport  Port=2  OutDataTypeStr=boolean  PortDimensions=1  SampleTime=1.62760416666667e-08
  Delay : Delay  DelayLength=DelayLength  InitialCondition=InitialCondition  ShowEnablePort=on
      settings: InputPortMap=u0,e6
  StateControl : StateControl  StateControl=Synchronous
  y : Outport  SampleTime=1.62760416666667e-08
  wires:
  Delay/1 -> y/1
  u/1 -> Delay/1
  E/1 -> Delay/2

== system gm_nrhdlSignalDetection/SSB Detect and Demod/PSS Detector/Find Peak/Delay Enabled Synchronous ==
  u : Inport  OutDataTypeStr=boolean  PortDimensions=1  SampleTime=1.62760416666667e-08
  E : Inport  Port=2  OutDataTypeStr=boolean  PortDimensions=1  SampleTime=1.62760416666667e-08
  Synchronous Delay : Subsystem
  y : Outport  SampleTime=1.62760416666667e-08
  wires:
  u/1 -> Synchronous Delay/1(u)
  E/1 -> Synchronous Delay/2(E)
  Synchronous Delay/1(y) -> y/1

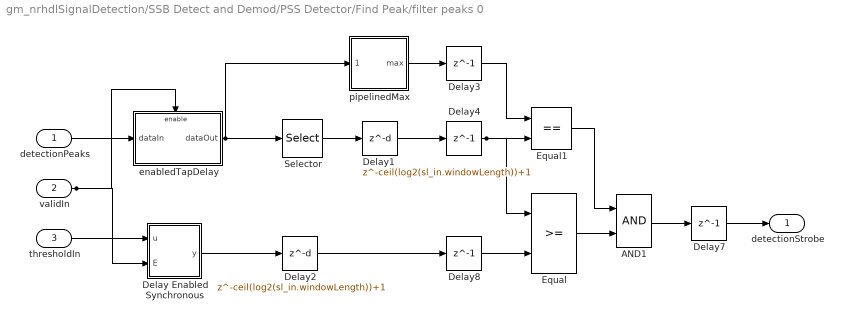
== system gm_nrhdlSignalDetection/SSB Detect and Demod/PSS Detector/Find Peak/filter peaks 0 ==
  detectionPeaks : Inport  OutDataTypeStr=fixdt(1, 36, 26)  PortDimensions=1  SampleTime=1.62760416666667e-08
  validIn : Inport  Port=2  OutDataTypeStr=boolean  PortDimensions=1  SampleTime=1.62760416666667e-08
  thresholdIn : Inport  Port=3  OutDataTypeStr=fixdt(0, 32, 24)  PortDimensions=1  SampleTime=1.62760416666667e-08
  AND1 : Logic  AllPortsSameDT=off  OutDataTypeStr=boolean
  Delay Enabled Synchronous : Subsystem  mask(Delay Enabled){DelayLength=ceil(sl_in.windowLength/2), InitialCondition=0.0}
      mask prompts: DelayLength "Simulink:blkprm_prompts:DelayBlkDelayLength"; InitialCondition "Simulink:blkprm_prompts:DelayBlkInitCond"
      mask help: Implements a delay with synchronous enable.
      mask Display:
      | port_label('input', 1, 'u');
      | port_label('input', 2, 'E');
      | text(0.45,0.45, 'Z');
      | DelayLengthStr = get_param(gcbh,'DelayLength');
      | try
      |     DelayLength = eval(DelayLengthStr);
      |     text(0.55,0.55, sprintf('-%d',DelayLength));
      | catch ME
      |     text(0.55,0.55, '-N');
      | end
  Delay1 : Delay  DelayLength=ceil(log2(sl_in.windowLength))+1
  Delay2 : Delay  DelayLength=ceil(log2(sl_in.windowLength))+1
  Delay3 : Delay  DelayLength=1
  Delay4 : Delay  DelayLength=1
  Delay7 : Delay  DelayLength=1
  Delay8 : Delay  DelayLength=1  InitialCondition=1
  Equal : RelationalOperator  OutDataTypeStr=boolean  RndMeth=Simplest  InputSameDT=off
  Equal1 : RelationalOperator  Operator===  OutDataTypeStr=boolean  RndMeth=Simplest  InputSameDT=off
  Selector : Selector  InputPortWidth=sl_in.windowLength  IndexOptions=Index vector (dialog)  Indices=ceil(sl_in.windowLength/2)  OutputSizes=1
  enabledTapDelay : Subsystem
  pipelinedMax : Subsystem
  detectionStrobe : Outport  SampleTime=1.62760416666667e-08
  wires:
  Delay1/1 -> Delay4/1
  Delay2/1 -> Delay8/1
  detectionPeaks/1 -> enabledTapDelay/1(dataIn)
  enabledTapDelay/1(dataOut) -> Selector/1, pipelinedMax/1(peaks)
  pipelinedMax/1(max) -> Delay3/1
  validIn/1 -> enabledTapDelay/Enable, Delay Enabled Synchronous/2(E)
  thresholdIn/1 -> Delay Enabled Synchronous/1(u)
  Delay Enabled Synchronous/1(y) -> Delay2/1
  Equal1/1 -> AND1/1
  Selector/1 -> Delay1/1
  Delay4/1 -> Equal1/2, Equal/1
  Delay3/1 -> Equal1/1
  Delay7/1 -> detectionStrobe/1
  Delay8/1 -> Equal/2
  Equal/1 -> AND1/2
  AND1/1 -> Delay7/1

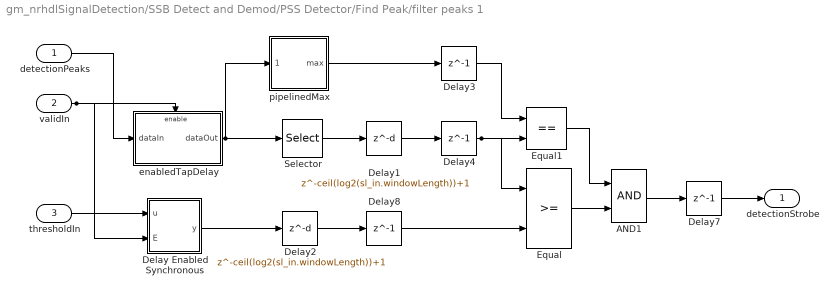
== system gm_nrhdlSignalDetection/SSB Detect and Demod/PSS Detector/Find Peak/filter peaks 1 ==
  detectionPeaks : Inport  OutDataTypeStr=fixdt(1, 36, 26)  PortDimensions=1  SampleTime=1.62760416666667e-08
  validIn : Inport  Port=2  OutDataTypeStr=boolean  PortDimensions=1  SampleTime=1.62760416666667e-08
  thresholdIn : Inport  Port=3  OutDataTypeStr=fixdt(0, 32, 24)  PortDimensions=1  SampleTime=1.62760416666667e-08
  AND1 : Logic  AllPortsSameDT=off  OutDataTypeStr=boolean
  Delay Enabled Synchronous : Subsystem  mask(Delay Enabled){DelayLength=ceil(sl_in.windowLength/2), InitialCondition=0.0}
      mask prompts: DelayLength "Simulink:blkprm_prompts:DelayBlkDelayLength"; InitialCondition "Simulink:blkprm_prompts:DelayBlkInitCond"
      mask help: Implements a delay with synchronous enable.
      mask Display:
      | port_label('input', 1, 'u');
      | port_label('input', 2, 'E');
      | text(0.45,0.45, 'Z');
      | DelayLengthStr = get_param(gcbh,'DelayLength');
      | try
      |     DelayLength = eval(DelayLengthStr);
      |     text(0.55,0.55, sprintf('-%d',DelayLength));
      | catch ME
      |     text(0.55,0.55, '-N');
      | end
  Delay1 : Delay  DelayLength=ceil(log2(sl_in.windowLength))+1
  Delay2 : Delay  DelayLength=ceil(log2(sl_in.windowLength))+1
  Delay3 : Delay  DelayLength=1
  Delay4 : Delay  DelayLength=1
  Delay7 : Delay  DelayLength=1
  Delay8 : Delay  DelayLength=1  InitialCondition=1
  Equal : RelationalOperator  OutDataTypeStr=boolean  RndMeth=Simplest  InputSameDT=off
  Equal1 : RelationalOperator  Operator===  OutDataTypeStr=boolean  RndMeth=Simplest  InputSameDT=off
  Selector : Selector  InputPortWidth=sl_in.windowLength  IndexOptions=Index vector (dialog)  Indices=ceil(sl_in.windowLength/2)  OutputSizes=1
  enabledTapDelay : Subsystem
  pipelinedMax : Subsystem
  detectionStrobe : Outport  SampleTime=1.62760416666667e-08
  wires:
  detectionPeaks/1 -> enabledTapDelay/1(dataIn)
  Delay2/1 -> Delay8/1
  validIn/1 -> Delay Enabled Synchronous/2(E), enabledTapDelay/Enable
  thresholdIn/1 -> Delay Enabled Synchronous/1(u)
  Delay Enabled Synchronous/1(y) -> Delay2/1
  enabledTapDelay/1(dataOut) -> Selector/1, pipelinedMax/1(peaks)
  pipelinedMax/1(max) -> Delay3/1
  Selector/1 -> Delay1/1
  Delay1/1 -> Delay4/1
  Delay8/1 -> Equal/2
  Delay3/1 -> Equal1/1
  Delay4/1 -> Equal1/2, Equal/1
  Equal1/1 -> AND1/1
  Equal/1 -> AND1/2
  AND1/1 -> Delay7/1
  Delay7/1 -> detectionStrobe/1

== system gm_nrhdlSignalDetection/SSB Detect and Demod/PSS Detector/Find Peak/filter peaks 2 ==
  detectionPeaks : Inport  OutDataTypeStr=fixdt(1, 36, 26)  PortDimensions=1  SampleTime=1.62760416666667e-08
  validIn : Inport  Port=2  OutDataTypeStr=boolean  PortDimensions=1  SampleTime=1.62760416666667e-08
  thresholdIn : Inport  Port=3  OutDataTypeStr=fixdt(0, 32, 24)  PortDimensions=1  SampleTime=1.62760416666667e-08
  AND1 : Logic  AllPortsSameDT=off  OutDataTypeStr=boolean
  Delay Enabled Synchronous : Subsystem  mask(Delay Enabled){DelayLength=ceil(sl_in.windowLength/2), InitialCondition=0.0}
      mask prompts: DelayLength "Simulink:blkprm_prompts:DelayBlkDelayLength"; InitialCondition "Simulink:blkprm_prompts:DelayBlkInitCond"
      mask help: Implements a delay with synchronous enable.
      mask Display:
      | port_label('input', 1, 'u');
      | port_label('input', 2, 'E');
      | text(0.45,0.45, 'Z');
      | DelayLengthStr = get_param(gcbh,'DelayLength');
      | try
      |     DelayLength = eval(DelayLengthStr);
      |     text(0.55,0.55, sprintf('-%d',DelayLength));
      | catch ME
      |     text(0.55,0.55, '-N');
      | end
  Delay1 : Delay  DelayLength=ceil(log2(sl_in.windowLength))+1
  Delay2 : Delay  DelayLength=ceil(log2(sl_in.windowLength))+1
  Delay3 : Delay  DelayLength=1
  Delay4 : Delay  DelayLength=1
  Delay7 : Delay  DelayLength=1
  Delay8 : Delay  DelayLength=1  InitialCondition=1
  Equal : RelationalOperator  OutDataTypeStr=boolean  RndMeth=Simplest  InputSameDT=off
  Equal1 : RelationalOperator  Operator===  OutDataTypeStr=boolean  RndMeth=Simplest  InputSameDT=off
  Selector : Selector  InputPortWidth=sl_in.windowLength  IndexOptions=Index vector (dialog)  Indices=ceil(sl_in.windowLength/2)  OutputSizes=1
  enabledTapDelay : Subsystem
  pipelinedMax : Subsystem
  detectionStrobe : Outport  SampleTime=1.62760416666667e-08
  wires:
  thresholdIn/1 -> Delay Enabled Synchronous/1(u)
  enabledTapDelay/1(dataOut) -> Selector/1, pipelinedMax/1(peaks)
  detectionPeaks/1 -> enabledTapDelay/1(dataIn)
  validIn/1 -> enabledTapDelay/Enable, Delay Enabled Synchronous/2(E)
  Delay Enabled Synchronous/1(y) -> Delay2/1
  pipelinedMax/1(max) -> Delay3/1
  Delay2/1 -> Delay8/1
  Selector/1 -> Delay1/1
  Delay1/1 -> Delay4/1
  Delay8/1 -> Equal/2
  Delay3/1 -> Equal1/1
  Delay4/1 -> Equal1/2, Equal/1
  Equal1/1 -> AND1/1
  Equal/1 -> AND1/2
  AND1/1 -> Delay7/1
  Delay7/1 -> detectionStrobe/1

== system gm_nrhdlSignalDetection/SSB Detect and Demod/PSS Detector/Find Peak/register PSS ID ==
  A : Inport  OutDataTypeStr=boolean  PortDimensions=1  SampleTime=1.62760416666667e-08
  B : Inport  Port=2  OutDataTypeStr=boolean  PortDimensions=1  SampleTime=1.62760416666667e-08
  C : Inport  Port=3  OutDataTypeStr=boolean  PortDimensions=1  SampleTime=1.62760416666667e-08
  validIn : Inport  Port=4  OutDataTypeStr=boolean  PortDimensions=1  SampleTime=1.62760416666667e-08
  start : Inport  Port=5  OutDataTypeStr=boolean  PortDimensions=1  SampleTime=1.62760416666667e-08
  register PSS ID : MATLAB Function  TreatAsAtomicUnit=on
  selectedPSS : Outport  SampleTime=1.62760416666667e-08
  valid : Outport  Port=2  SampleTime=1.62760416666667e-08
  wires:
  A/1 -> register PSS ID/1(A)
  B/1 -> register PSS ID/2(B)
  C/1 -> register PSS ID/3(C)
  register PSS ID/1(selectedPSS) -> selectedPSS/1
  validIn/1 -> register PSS ID/4(validIn)
  start/1 -> register PSS ID/5(start)
  register PSS ID/2(valid) -> valid/1

== system gm_nrhdlSignalDetection/SSB Detect and Demod/PSS Detector/Stream Synchronizer/MATLAB Function ==
  pop : Inport  OutDataTypeStr=boolean  PortDimensions=1  SampleTime=1.62760416666667e-08
  push : Inport  Port=2  OutDataTypeStr=boolean  PortDimensions=1  SampleTime=1.62760416666667e-08
  MATLAB Function : MATLAB Function  InitFcn=Simulink.suppressDiagnostic(gcb, 'Stateflow:Runtime:DataOverflowErrorMSLD');  TreatAsAtomicUnit=on
  wrAddr : Outport  SampleTime=1.62760416666667e-08
  wrEn : Outport  Port=2  SampleTime=1.62760416666667e-08
  rdAddr : Outport  Port=3  SampleTime=1.62760416666667e-08
  validOut : Outport  Port=4  SampleTime=1.62760416666667e-08
  wires:
  pop/1 -> MATLAB Function/1(pop)
  MATLAB Function/4(validOut) -> validOut/1
  push/1 -> MATLAB Function/2(push)
  MATLAB Function/1(wrAddr) -> wrAddr/1
  MATLAB Function/3(rdAddr) -> rdAddr/1
  MATLAB Function/2(wrEn) -> wrEn/1

== system gm_nrhdlSignalDetection/SSB Detect and Demod/PSS Detector/signalMagAverage/Synchronous Enabled Nfft Sample Delay  ==
  dataIn : Inport  OutDataTypeStr=fixdt(0, 43, 34)  PortDimensions=1  SampleTime=1.62760416666667e-08
  en : Inport  Port=2  OutDataTypeStr=boolean  PortDimensions=1  SampleTime=1.62760416666667e-08
  Delay1 : Delay  DelayLength=sl_in.Nfft  InitialCondition=0  ShowEnablePort=on
      settings: InputPortMap=u0,e6
  StateControl : StateControl  StateControl=Synchronous
  dataOut : Outport  SampleTime=1.62760416666667e-08  VectorParamsAs1DForOutWhenUnconnected=off
  wires:
  dataIn/1 -> Delay1/1
  en/1 -> Delay1/2
  Delay1/1 -> dataOut/1

== system gm_nrhdlSignalDetection/SSB Detect and Demod/PSS Detector/Find Peak/Delay Enabled Synchronous/Synchronous Delay ==
  u : Inport  OutDataTypeStr=boolean  PortDimensions=1  SampleTime=1.62760416666667e-08
  E : Inport  Port=2  OutDataTypeStr=boolean  PortDimensions=1  SampleTime=1.62760416666667e-08
  Delay : Delay  DelayLength=DelayLength  InitialCondition=InitialCondition  ShowEnablePort=on
      settings: InputPortMap=u0,e6
  StateControl : StateControl  StateControl=Synchronous
  y : Outport  SampleTime=1.62760416666667e-08
  wires:
  u/1 -> Delay/1
  E/1 -> Delay/2
  Delay/1 -> y/1

== system gm_nrhdlSignalDetection/SSB Detect and Demod/PSS Detector/Find Peak/filter peaks 0/Delay Enabled Synchronous ==
  u : Inport  OutDataTypeStr=fixdt(0, 32, 24)  PortDimensions=1  SampleTime=1.62760416666667e-08
  E : Inport  Port=2  OutDataTypeStr=boolean  PortDimensions=1  SampleTime=1.62760416666667e-08
  Synchronous Delay : Subsystem
  y : Outport  SampleTime=1.62760416666667e-08
  wires:
  u/1 -> Synchronous Delay/1(u)
  E/1 -> Synchronous Delay/2(E)
  Synchronous Delay/1(y) -> y/1

== system gm_nrhdlSignalDetection/SSB Detect and Demod/PSS Detector/Find Peak/filter peaks 0/enabledTapDelay ==
  dataIn : Inport  OutDataTypeStr=fixdt(1, 36, 26)  PortDimensions=1  SampleTime=1.62760416666667e-08
  Enable : EnablePort  OutDataTypeStr=boolean
  StateControl : StateControl  StateControl=Synchronous
  Tapped Delay : simulink/Discrete/Tapped Delay  vinit=0.0  samptime=-1  NumDelays=sl_in.windowLength  DelayOrder=Oldest  includeCurrent=off
  dataOut : Outport  SampleTime=1.62760416666667e-08  InitialOutput=0
  wires:
  dataIn/1 -> Tapped Delay/1
  Tapped Delay/1 -> dataOut/1

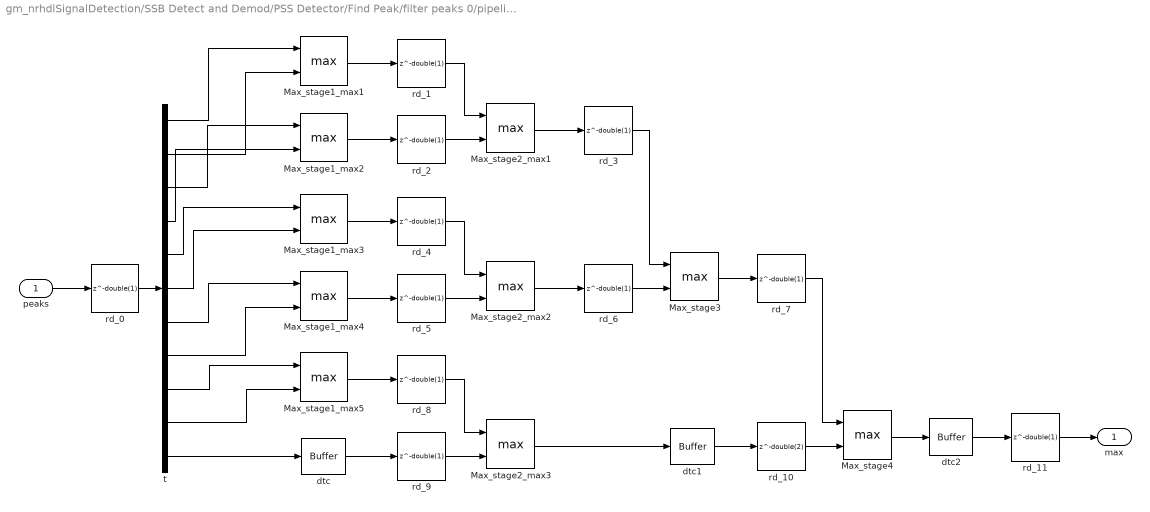
== system gm_nrhdlSignalDetection/SSB Detect and Demod/PSS Detector/Find Peak/filter peaks 0/pipelinedMax ==
  peaks : Inport  OutDataTypeStr=fixdt(1, 36, 26)  PortDimensions=[11]  SampleTime=1.62760416666667e-08
  Max_stage1_max{1..5} (5 alike) : MinMax  Function=max  Inputs=2
  Max_stage2_max1 : MinMax  Function=max  Inputs=2
  Max_stage2_max2 : MinMax  Function=max  Inputs=2
  Max_stage2_max3 : MinMax  Function=max  Inputs=2
  Max_stage3 : MinMax  Function=max  Inputs=2
  Max_stage4 : MinMax  Function=max  Inputs=2
  dtc : hdlmdlgenlib/Buffer
  dtc1 : hdlmdlgenlib/Buffer
  dtc2 : hdlmdlgenlib/Buffer
  rd_{0..9,11} (11 alike) : Delay  DelayLength=double(1)  InitialCondition=0  SampleTime=1.62760416666667e-08
  rd_10 : Delay  DelayLength=double(2)  InitialCondition=0  SampleTime=1.62760416666667e-08
  t : Demux  Outputs=11
  max : Outport  SampleTime=1.62760416666667e-08
  wires:
  Max_stage1_max1/1 -> rd_1/1
  peaks/1 -> rd_0/1
  dtc2/1 -> rd_11/1
  rd_0/1 -> t/1
  rd_9/1 -> Max_stage2_max3/2
  t/1 -> Max_stage1_max1/1
  t/2 -> Max_stage1_max1/2
  t/3 -> Max_stage1_max2/1
  t/4 -> Max_stage1_max2/2
  t/5 -> Max_stage1_max3/1
  t/6 -> Max_stage1_max3/2
  t/10 -> Max_stage1_max5/2
  t/9 -> Max_stage1_max5/1
  t/8 -> Max_stage1_max4/2
  t/7 -> Max_stage1_max4/1
  t/11 -> dtc/1
  Max_stage1_max2/1 -> rd_2/1
  Max_stage1_max3/1 -> rd_4/1
  Max_stage1_max5/1 -> rd_8/1
  Max_stage1_max4/1 -> rd_5/1
  dtc1/1 -> rd_10/1
  dtc/1 -> rd_9/1
  rd_1/1 -> Max_stage2_max1/1
  rd_11/1 -> max/1
  rd_2/1 -> Max_stage2_max1/2
  rd_3/1 -> Max_stage3/1
  rd_4/1 -> Max_stage2_max2/1
  rd_6/1 -> Max_stage3/2
  rd_5/1 -> Max_stage2_max2/2
  rd_7/1 -> Max_stage4/1
  rd_8/1 -> Max_stage2_max3/1
  Max_stage2_max1/1 -> rd_3/1
  Max_stage2_max2/1 -> rd_6/1
  rd_10/1 -> Max_stage4/2
  Max_stage3/1 -> rd_7/1
  Max_stage2_max3/1 -> dtc1/1
  Max_stage4/1 -> dtc2/1

== system gm_nrhdlSignalDetection/SSB Detect and Demod/PSS Detector/Find Peak/filter peaks 1/Delay Enabled Synchronous ==
  u : Inport  OutDataTypeStr=fixdt(0, 32, 24)  PortDimensions=1  SampleTime=1.62760416666667e-08
  E : Inport  Port=2  OutDataTypeStr=boolean  PortDimensions=1  SampleTime=1.62760416666667e-08
  Synchronous Delay : Subsystem
  y : Outport  SampleTime=1.62760416666667e-08
  wires:
  E/1 -> Synchronous Delay/2(E)
  u/1 -> Synchronous Delay/1(u)
  Synchronous Delay/1(y) -> y/1

== system gm_nrhdlSignalDetection/SSB Detect and Demod/PSS Detector/Find Peak/filter peaks 1/enabledTapDelay ==
  dataIn : Inport  OutDataTypeStr=fixdt(1, 36, 26)  PortDimensions=1  SampleTime=1.62760416666667e-08
  Enable : EnablePort  OutDataTypeStr=boolean
  StateControl : StateControl  StateControl=Synchronous
  Tapped Delay : simulink/Discrete/Tapped Delay  vinit=0.0  samptime=-1  NumDelays=sl_in.windowLength  DelayOrder=Oldest  includeCurrent=off
  dataOut : Outport  SampleTime=1.62760416666667e-08  InitialOutput=0
  wires:
  dataIn/1 -> Tapped Delay/1
  Tapped Delay/1 -> dataOut/1

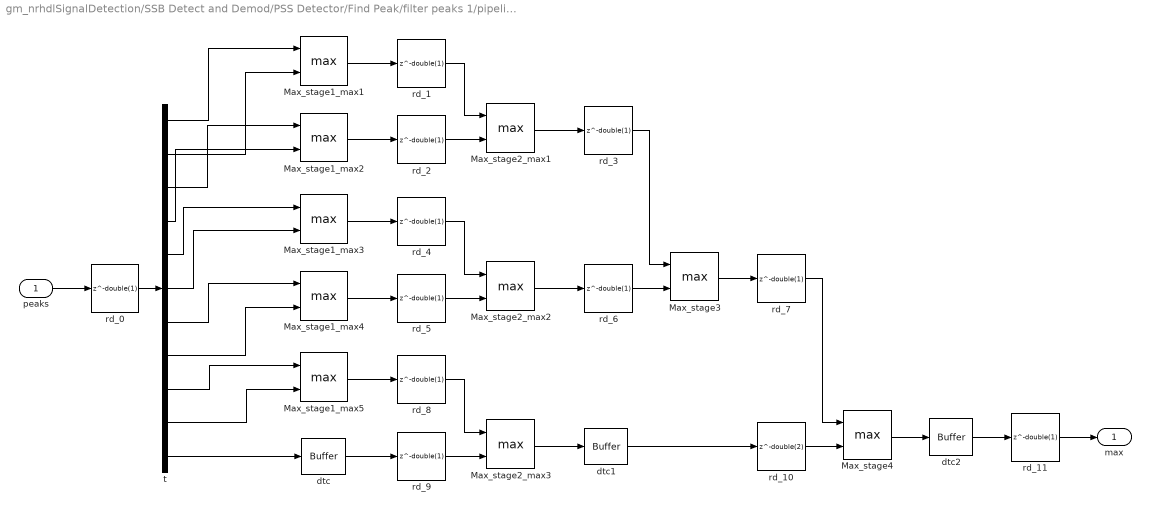
== system gm_nrhdlSignalDetection/SSB Detect and Demod/PSS Detector/Find Peak/filter peaks 1/pipelinedMax ==
  peaks : Inport  OutDataTypeStr=fixdt(1, 36, 26)  PortDimensions=[11]  SampleTime=1.62760416666667e-08
  Max_stage1_max{1..5} (5 alike) : MinMax  Function=max  Inputs=2
  Max_stage2_max1 : MinMax  Function=max  Inputs=2
  Max_stage2_max2 : MinMax  Function=max  Inputs=2
  Max_stage2_max3 : MinMax  Function=max  Inputs=2
  Max_stage3 : MinMax  Function=max  Inputs=2
  Max_stage4 : MinMax  Function=max  Inputs=2
  dtc : hdlmdlgenlib/Buffer
  dtc1 : hdlmdlgenlib/Buffer
  dtc2 : hdlmdlgenlib/Buffer
  rd_{0..9,11} (11 alike) : Delay  DelayLength=double(1)  InitialCondition=0  SampleTime=1.62760416666667e-08
  rd_10 : Delay  DelayLength=double(2)  InitialCondition=0  SampleTime=1.62760416666667e-08
  t : Demux  Outputs=11
  max : Outport  SampleTime=1.62760416666667e-08
  wires:
  t/1 -> Max_stage1_max1/1
  t/2 -> Max_stage1_max1/2
  rd_11/1 -> max/1
  peaks/1 -> rd_0/1
  t/3 -> Max_stage1_max2/1
  rd_0/1 -> t/1
  Max_stage2_max3/1 -> dtc1/1
  t/4 -> Max_stage1_max2/2
  t/5 -> Max_stage1_max3/1
  Max_stage3/1 -> rd_7/1
  t/6 -> Max_stage1_max3/2
  t/7 -> Max_stage1_max4/1
  t/8 -> Max_stage1_max4/2
  t/9 -> Max_stage1_max5/1
  t/10 -> Max_stage1_max5/2
  t/11 -> dtc/1
  Max_stage1_max1/1 -> rd_1/1
  Max_stage1_max2/1 -> rd_2/1
  rd_3/1 -> Max_stage3/1
  Max_stage1_max3/1 -> rd_4/1
  Max_stage1_max4/1 -> rd_5/1
  rd_5/1 -> Max_stage2_max2/2
  Max_stage1_max5/1 -> rd_8/1
  dtc/1 -> rd_9/1
  rd_1/1 -> Max_stage2_max1/1
  rd_2/1 -> Max_stage2_max1/2
  rd_4/1 -> Max_stage2_max2/1
  rd_8/1 -> Max_stage2_max3/1
  rd_9/1 -> Max_stage2_max3/2
  Max_stage2_max1/1 -> rd_3/1
  Max_stage2_max2/1 -> rd_6/1
  rd_6/1 -> Max_stage3/2
  dtc1/1 -> rd_10/1
  rd_7/1 -> Max_stage4/1
  rd_10/1 -> Max_stage4/2
  Max_stage4/1 -> dtc2/1
  dtc2/1 -> rd_11/1

== system gm_nrhdlSignalDetection/SSB Detect and Demod/PSS Detector/Find Peak/filter peaks 2/Delay Enabled Synchronous ==
  u : Inport  OutDataTypeStr=fixdt(0, 32, 24)  PortDimensions=1  SampleTime=1.62760416666667e-08
  E : Inport  Port=2  OutDataTypeStr=boolean  PortDimensions=1  SampleTime=1.62760416666667e-08
  Synchronous Delay : Subsystem
  y : Outport  SampleTime=1.62760416666667e-08
  wires:
  Synchronous Delay/1(y) -> y/1
  u/1 -> Synchronous Delay/1(u)
  E/1 -> Synchronous Delay/2(E)

== system gm_nrhdlSignalDetection/SSB Detect and Demod/PSS Detector/Find Peak/filter peaks 2/enabledTapDelay ==
  dataIn : Inport  OutDataTypeStr=fixdt(1, 36, 26)  PortDimensions=1  SampleTime=1.62760416666667e-08
  Enable : EnablePort  OutDataTypeStr=boolean
  StateControl : StateControl  StateControl=Synchronous
  Tapped Delay : simulink/Discrete/Tapped Delay  vinit=0.0  samptime=-1  NumDelays=sl_in.windowLength  DelayOrder=Oldest  includeCurrent=off
  dataOut : Outport  SampleTime=1.62760416666667e-08  InitialOutput=0
  wires:
  dataIn/1 -> Tapped Delay/1
  Tapped Delay/1 -> dataOut/1
